simulink model "func_mov_avg"  (R2024a)
settings: configuration reference "SharedConfig" (kept outside this file)
libraries: simulink x1
settings Model: DataDictionary=configuration_dictionary.sldd  Creator=matlab.cut  LastModifiedBy=matlab.cut
settings ConfigSetRef: SourceName=SharedConfig

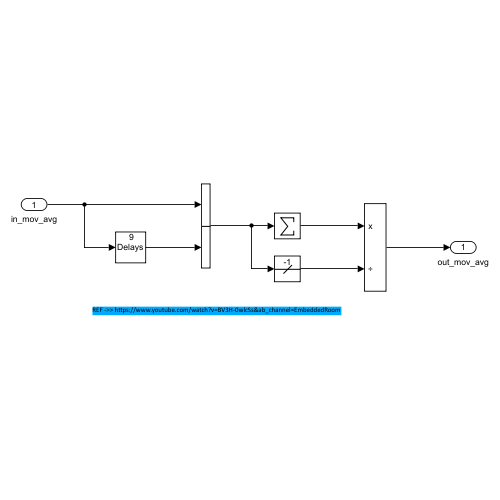
[thumbnail: Simulink's stored preview of the top-level diagram]
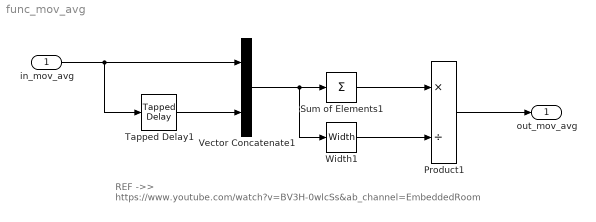
== system func_mov_avg ==
  note: REF ->> https://www.youtube.com/watch?v=BV3H-0wlcSs&ab_channel=EmbeddedRoom
  in_mov_avg : Inport
  Product1 : Product  Inputs=*/
  Sum of Elements1 : Sum  Inputs=+
  Tapped Delay1 : simulink/Discrete/Tapped Delay  vinit=0  samptime=-1  NumDelays=9  DelayOrder=Oldest  includeCurrent=off
  Vector Concatenate1 : Concatenate
  Width1 : Width
  out_mov_avg : Outport
  wires:
  Vector Concatenate1/1 -> Sum of Elements1/1, Width1/1
  Tapped Delay1/1 -> Vector Concatenate1/2
  Sum of Elements1/1 -> Product1/1
  Product1/1 -> out_mov_avg/1
  in_mov_avg/1 -> Vector Concatenate1/1, Tapped Delay1/1
  Width1/1 -> Product1/2
